simulink model "vodorod"  (R2018b)
settings: Solver=FixedStepAuto  StartTime=0.0  StopTime=2  RelTol=1e-3
undefined symbols (not defined in the file): DiscIntNeverNeededParam
libraries: powerlib x17, simulink x1, simulink_extras x1
settings Model: Creator=Anton  LastModifiedBy=sr1
settings SFSimCC: SimUseLocalCustomCode=off
settings RTWCC: RTWUseLocalCustomCode=off
settings CodeAppCC: StateflowObjectComments=on
settings SimscapeCC: SimscapeNormalizeSystem=off

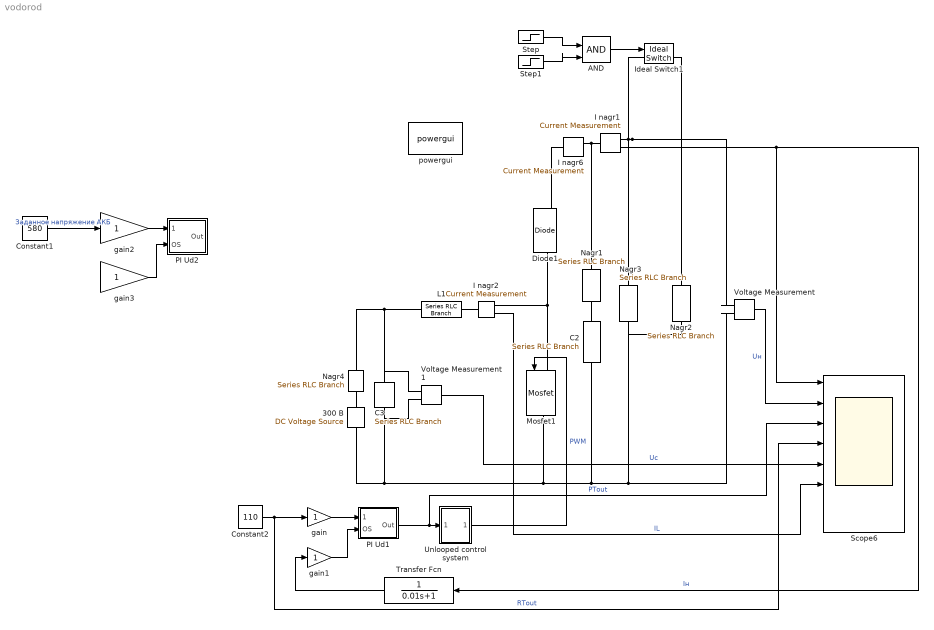
== system vodorod ==
  300 В : powerlib/Electrical Sources/DC Voltage Source  Amplitude=300  Measurements=None
      settings: SourceProductName=Simscape Electrical
  AND : Logic  IconShape=distinctive  AllPortsSameDT=off  OutDataTypeStr=boolean
  C2 : powerlib/Elements/Series RLC Branch  LConnTagsString=__new0  RConnTagsString=__new0  BranchType=C  Resistance=1e-6  Inductance=1e-3  SetiL0=off  InitialCurrent=0  Capacitance=8e-3  Setx0=on  InitialVoltage=400  Measurements=Branch voltage
      settings: SourceProductName=Simscape Electrical
  C3 : powerlib/Elements/Series RLC Branch  LConnTagsString=__new0  RConnTagsString=__new0  BranchType=C  Resistance=1e-6  Inductance=1e-3  SetiL0=off  InitialCurrent=0  Capacitance=8e-3  Setx0=on  InitialVoltage=320  Measurements=Branch voltage
      settings: SourceProductName=Simscape Electrical
  Constant1 : Constant  Value=580
  Constant2 : Constant  Value=110
  Diode1 : powerlib/Power Electronics/Diode  Ron=0.001  Lon=0  Vf=0.8  IC=0  UseSnubber=off  Rs=500  Cs=250e-9  Measurements=on
      settings: SourceProductName=Simscape Electrical
  I nagr1 : powerlib/Measurements/Current Measurement  PhasorSimulation=off  OutputType=Complex  PSBequivalent=0
      settings: SourceProductName=Simscape Electrical
  I nagr2 : powerlib/Measurements/Current Measurement  PhasorSimulation=off  OutputType=Complex  PSBequivalent=0
      settings: SourceProductName=Simscape Electrical
  I nagr6 : powerlib/Measurements/Current Measurement  PhasorSimulation=off  OutputType=Complex  PSBequivalent=0
      settings: SourceProductName=Simscape Electrical
  Ideal Switch1 : powerlib/Power Electronics/Ideal Switch  Ron=550*550/45000  Lon=0  IC=0  Rs=1e5  Cs=inf  Measurements=on
  L1 : powerlib/Elements/Series RLC Branch  LConnTagsString=__new0  RConnTagsString=__new0  BranchType=RL  Resistance=0.083  Inductance=0.82e-3  SetiL0=off  InitialCurrent=0  Capacitance=1e-6  Setx0=off  InitialVoltage=0  Measurements=None
      settings: SourceProductName=Simscape Electrical
  Mosfet1 : powerlib/Power Electronics/Mosfet  Ron=1e-6  Lon=0  Rd=1e-6  Vfd=0  IC=0  Rs=1e5  Cs=inf  Measurements=off
      settings: SourceProductName=Simscape Electrical
  Nagr1 : powerlib/Elements/Series RLC Branch  LConnTagsString=__new0  RConnTagsString=__new0  BranchType=R  Resistance=0.05  Inductance=1e-3  SetiL0=off  InitialCurrent=0  Capacitance=1e-6  Setx0=off  InitialVoltage=0  Measurements=None
      settings: SourceProductName=Simscape Electrical
  Nagr2 : powerlib/Elements/Series RLC Branch  LConnTagsString=__new0  RConnTagsString=__new0  BranchType=R  Resistance=40  Inductance=1e-3  SetiL0=off  InitialCurrent=0  Capacitance=1e-6  Setx0=off  InitialVoltage=0  Measurements=None
      settings: SourceProductName=Simscape Electrical
  Nagr3 : powerlib/Elements/Series RLC Branch  LConnTagsString=__new0  RConnTagsString=__new0  BranchType=R  Resistance=5  Inductance=1e-3  SetiL0=off  InitialCurrent=0  Capacitance=1e-6  Setx0=off  InitialVoltage=0  Measurements=None
      settings: SourceProductName=Simscape Electrical
  Nagr4 : powerlib/Elements/Series RLC Branch  LConnTagsString=__new0  RConnTagsString=__new0  BranchType=R  Resistance=0.15  Inductance=1e-3  SetiL0=off  InitialCurrent=0  Capacitance=1e-6  Setx0=off  InitialVoltage=0  Measurements=None
      settings: SourceProductName=Simscape Electrical
  PI Ud1 : Subsystem
  PI Ud2 : Subsystem
  Scope6 : Scope  NumInputPorts=8
  Step : Step  Time=0.5  SampleTime=0
  Step1 : Step  Before=1  After=0  SampleTime=0
  Transfer Fcn : TransferFcn  Denominator=[0.01 1]
  Unlooped control system : Subsystem
  Voltage Measurement : powerlib/Measurements/Voltage Measurement  PhasorSimulation=off  OutputType=Complex  PSBequivalent=0
  Voltage Measurement1 : powerlib/Measurements/Voltage Measurement  PhasorSimulation=off  OutputType=Complex  PSBequivalent=0
  gain{,1..3} (4 alike) : Gain  SaturateOnIntegerOverflow=on  OutDataTypeStr=Inherit: Same as input  ParamDataTypeStr=Inherit: Same as input
  powergui : powerlib/powergui  Priority=1  SimulationMode=Discrete  SampleTime=1e-6  frequency=60  Iterations=50  frequencyindice=0  Pbase=100e6  ErrMax=1e-4  UnitsV=kV  UnitsW=MW  buscounter=0  FunctionMessages=off  echomessages=off  EnableUseOfTLC=off  CurrentSourceSwitches=off  DisableSnubberDevices=off  DisableRonSwitches=off  DisableVfSwitches=off  DisplayEquations=off  SolverType=Tustin/Backward Euler (TBE)  Interpol=off  ExternalGateDelay=off  methode=off  Ts=100  x0status=blocks  SPID=off  SwTol=0  HookPort=off  RestoreLinks=warning  ResistiveCurrentMeasurement=off  Frange=[0:2:500]  Ylog=off  Xlog=on  ShowGrid=off  save=off  variable=ZData  structure=0  ZoomFFT=off  StartTime=0.0  cycles=1  DisplayStyle=1  fundamental=60  FreqAxis=off  MaxFrequency=1000  frequencyindicesteady=1  RmsSteady=1  display=off
  wires:
  gain/1 -> PI Ud1/1(Zad)
  gain1/1 -> PI Ud1/2(OS)
  PI Ud1/1(Out) -> Unlooped control system/1(Uz), Scope6/3  "РТout"
  gain3/1 -> PI Ud2/2(OS)
  Constant1/1 -> gain2/1  "Заданное напряжение АКБ"
  gain2/1 -> PI Ud2/1(Zad)
  Constant2/1 -> gain/1, Scope6/4  "RTout"
  Transfer Fcn/1 -> gain1/1
  Voltage Measurement/1 -> Scope6/2  "Uн"
  I nagr1/1 -> Transfer Fcn/1, Scope6/1  "Iн"
  Unlooped control system/1(CH1) -> Mosfet1/1  "PWM"
  Step/1 -> AND/1
  Step1/1 -> AND/2
  AND/1 -> Ideal Switch1/1
  Voltage Measurement1/1 -> Scope6/5  "Uc"
  I nagr2/1 -> Scope6/6  "IL"
  connections:
  Mosfet1/RConn1 -- Nagr2/RConn1 -- Nagr3/RConn1 -- Voltage Measurement/LConn2 -- C2/RConn1 -- Voltage Measurement1/LConn2 -- C3/RConn1 -- 300 В/LConn1
  Nagr4/RConn1 -- 300 В/RConn1
  Nagr4/LConn1 -- Voltage Measurement1/LConn1 -- C3/LConn1 -- L1/LConn1
  Mosfet1/LConn1 -- Diode1/LConn1 -- I nagr2/RConn1
  C2/LConn1 -- Nagr1/RConn1
  I nagr2/LConn1 -- L1/RConn1
  I nagr6/LConn1 -- Diode1/RConn1
  I nagr6/RConn1 -- I nagr1/LConn1 -- Nagr1/LConn1
  Nagr3/LConn1 -- Ideal Switch1/LConn1 -- Voltage Measurement/LConn1 -- I nagr1/RConn1
  Nagr2/LConn1 -- Ideal Switch1/RConn1

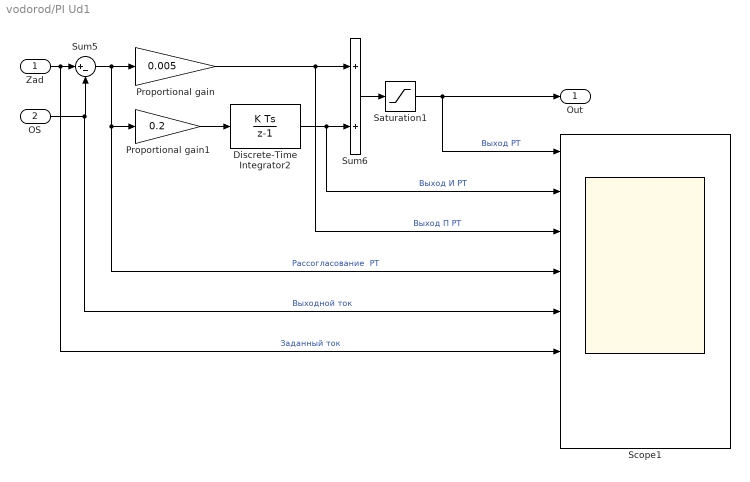
== system vodorod/PI Ud1 ==
  Zad : Inport
  OS : Inport  Port=2
  Discrete-Time Integrator2 : DiscreteIntegrator  SampleTime=-1  LimitOutput=on  UpperSaturationLimit=1  LowerSaturationLimit=0  ICPrevOutput=DiscIntNeverNeededParam  ICPrevScaledInput=DiscIntNeverNeededParam
  Proportional gain : Gain  Gain=0.005  SaturateOnIntegerOverflow=on  OutDataTypeStr=Inherit: Same as input  ParamDataTypeStr=Inherit: Same as input
  Proportional gain1 : Gain  Gain=0.2  SaturateOnIntegerOverflow=on  OutDataTypeStr=Inherit: Same as input  ParamDataTypeStr=Inherit: Same as input
  Saturation1 : Saturate  UpperLimit=0.68  LowerLimit=0
  Scope1 : Scope  NumInputPorts=8
  Sum5 : Sum  Inputs=|+-  SaturateOnIntegerOverflow=on  InputSameDT=on  OutDataTypeStr=Inherit: Same as first input
  Sum6 : Sum  SaturateOnIntegerOverflow=on  InputSameDT=on  OutDataTypeStr=Inherit: Same as first input
  Out : Outport
  wires:
  Proportional gain/1 -> Scope1/3, Sum6/1  "Выход П РТ"
  Discrete-Time Integrator2/1 -> Sum6/2, Scope1/2  "Выход И РТ"
  OS/1 -> Scope1/5, Sum5/2  "Выходной ток"
  Zad/1 -> Scope1/6, Sum5/1  "Заданный ток"
  Sum5/1 -> Proportional gain1/1, Scope1/4, Proportional gain/1  "Рассогласование  РТ"
  Sum6/1 -> Saturation1/1
  Saturation1/1 -> Out/1, Scope1/1  "Выход РТ"
  Proportional gain1/1 -> Discrete-Time Integrator2/1

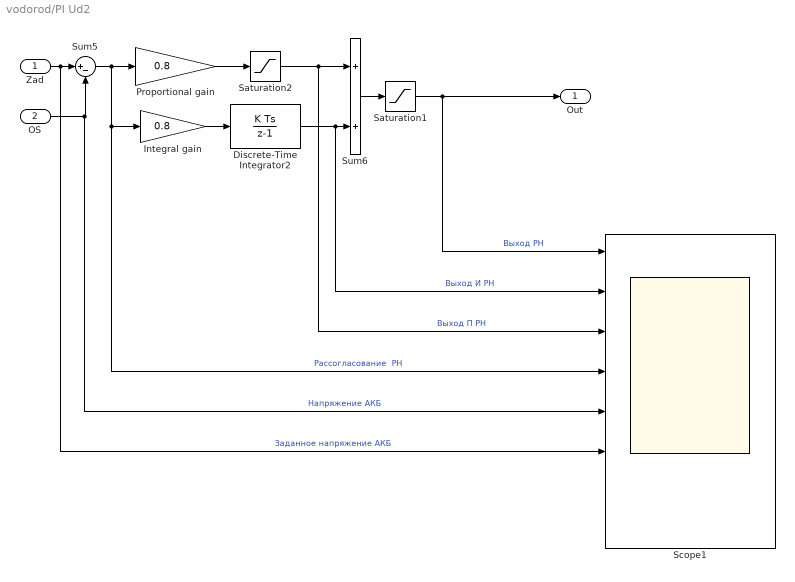
== system vodorod/PI Ud2 ==
  Zad : Inport
  OS : Inport  Port=2
  Discrete-Time Integrator2 : DiscreteIntegrator  SampleTime=-1  LimitOutput=on  UpperSaturationLimit=80  LowerSaturationLimit=0  ICPrevOutput=DiscIntNeverNeededParam  ICPrevScaledInput=DiscIntNeverNeededParam
  Integral gain : Gain  Gain=0.8  SaturateOnIntegerOverflow=on  OutDataTypeStr=Inherit: Same as input  ParamDataTypeStr=Inherit: Same as input
  Proportional gain : Gain  Gain=0.8  SaturateOnIntegerOverflow=on  OutDataTypeStr=Inherit: Same as input  ParamDataTypeStr=Inherit: Same as input
  Saturation1 : Saturate  UpperLimit=25  LowerLimit=0
  Saturation2 : Saturate  UpperLimit=1  LowerLimit=-1
  Scope1 : Scope  NumInputPorts=8
  Sum5 : Sum  Inputs=|+-  SaturateOnIntegerOverflow=on  InputSameDT=on  OutDataTypeStr=Inherit: Same as first input
  Sum6 : Sum  SaturateOnIntegerOverflow=on  InputSameDT=on  OutDataTypeStr=Inherit: Same as first input
  Out : Outport
  wires:
  Integral gain/1 -> Discrete-Time Integrator2/1
  Discrete-Time Integrator2/1 -> Scope1/2, Sum6/2  "Выход И РН"
  OS/1 -> Scope1/5, Sum5/2  "Напряжение АКБ"
  Zad/1 -> Scope1/6, Sum5/1  "Заданное напряжение АКБ"
  Sum5/1 -> Scope1/4, Integral gain/1, Proportional gain/1  "Рассогласование  РН"
  Sum6/1 -> Saturation1/1
  Saturation1/1 -> Out/1, Scope1/1  "Выход РН"
  Proportional gain/1 -> Saturation2/1
  Saturation2/1 -> Scope1/3, Sum6/1  "Выход П РН"

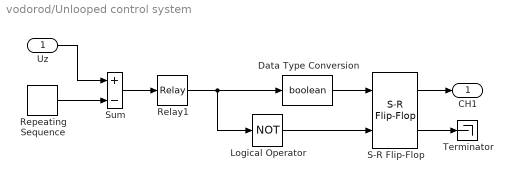
== system vodorod/Unlooped control system ==
  Uz : Inport
  Data Type Conversion : DataTypeConversion  OutDataTypeStr=boolean
  Logical Operator : Logic  Operator=NOT  AllPortsSameDT=off  OutDataTypeStr=boolean
  Relay1 : Relay  OnSwitchValue=0.01  OffSwitchValue=-0.01
  Repeating Sequence : simulink/Sources/Repeating Sequence  rep_seq_t="[0  0.000125 0.00025]"  rep_seq_y=[0 1 0]
  S-R Flip-Flop : simulink_extras/Flip Flops/S-R Flip-Flop  initial_condition=0
  Sum : Sum  Inputs=+-
  Terminator : Terminator
  CH1 : Outport
  wires:
  S-R Flip-Flop/1 -> CH1/1
  Data Type Conversion/1 -> S-R Flip-Flop/1
  Logical Operator/1 -> S-R Flip-Flop/2
  Relay1/1 -> Logical Operator/1, Data Type Conversion/1
  Repeating Sequence/1 -> Sum/2
  Uz/1 -> Sum/1
  Sum/1 -> Relay1/1
  S-R Flip-Flop/2 -> Terminator/1
